simulink model "motor_model"  (R2025b)
settings: Solver=VariableStepAuto  StartTime=0.0  StopTime=10.0  RelTol=1e-3
settings Model: Creator=abirp  LastModifiedBy=abirp

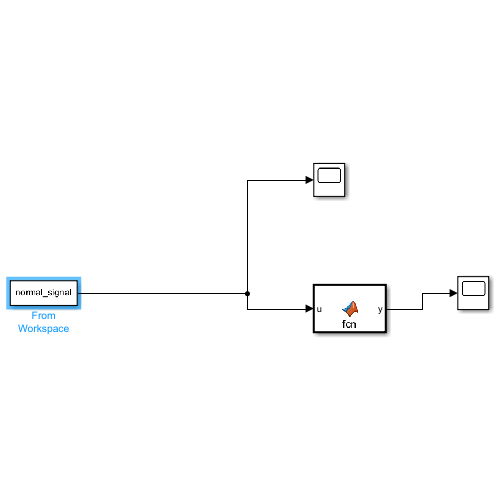
[thumbnail: Simulink's stored preview of the top-level diagram]
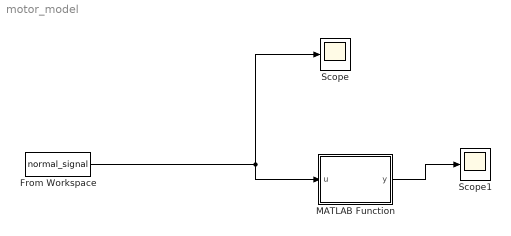
== system motor_model ==
  From Workspace : FromWorkspace  VariableName=normal_signal
  MATLAB Function : MATLAB Function  TreatAsAtomicUnit=on
  Scope : Scope
      settings: ActiveDisplayYMinimum=-0.36137399999964354  ActiveDisplayYMaximum=0.3859906153845758
  Scope1 : Scope
      settings: ActiveDisplayYMinimum=-0.038906769230769224  ActiveDisplayYMaximum=0.35016092307692309
  wires:
  From Workspace/1 -> MATLAB Function/1(u), Scope/1
  MATLAB Function/1(y) -> Scope1/1

== matlab function motor_model/MATLAB Function ==
  settings: updateMethod=DISCRETE  sampleTime=1/12000
  data: u input; y output
function y = fcn(u)
%#codegen

env = abs(hilbert(u));

N = length(env);
Y = fft(env);

P2 = abs(Y/N);
P1 = P2(1:N/2+1);
P1(2:end-1) = 2*P1(2:end-1);

y = P1(:);
end
